simulink model "TwoSegmentArm_muscles"  (R2024b)
settings: Solver=VariableStepAuto  StartTime=0.0  StopTime=5  RelTol=1e-3  AbsTol=1e-3  EnableMultiTasking=on
model workspace (MAT data in the model file):
  bp_out = [-2.4 1.9]
values from neighbouring files (symbols this model uses):
  Param_Mus_MEE = Library_mtu_simulink_mtu_standard_parameters(Param_Mus_MEE)    [init_muscle_MEE.m]
  Param_Mus_MEF = Library_mtu_simulink_mtu_standard_parameters(Param_Mus_MEF)    [init_muscle_MEF.m]
  Param_Mus_MSA = Library_mtu_simulink_mtu_standard_parameters(Param_Mus_MSA)    [init_muscle_MSA.m]
  Param_Mus_MSR = Library_mtu_simulink_mtu_standard_parameters(Param_Mus_MSR)    [init_muscle_MSR.m]
  random_offset = 0    [ddpg_agent.m]
  Ts = 0.075    [ddpg_agent.m]
undefined symbols (not defined in the file or in its folder): DiscIntNeverNeededParam, gaussian, X, Y, Z
libraries: sm_lib x25, nesl_utility x15, simulink x10, Library_mtu_simulink x8, rllib x1
(part 1 of 2)
settings Model: Creator=Isabell  LastModifiedBy=morit
settings SolverCC: AutoScaleAbsTol=off  AlgebraicLoopSolver=TrustRegion
settings DataIOCC: LimitDataPoints=on  MaxDataPoints=10000
settings OptimizationCC: LifeSpan=inf
settings DebuggingCC: UnconnectedInputMsg=warning  UnconnectedOutputMsg=warning  UnconnectedLineMsg=warning  AllowSymbolicDim=off  SFUnexpectedBacktrackingDiag=warning  SFNoUnconditionalDefaultTransitionDiag=warning  SFExecutionAtInitializationDiag=none  ArithmeticOperatorsInVariantConditions=warning
settings ModelReferenceCC: EnableRefExpFcnMdlSchedulingChecks=on
settings SFSimCC: SimUseLocalCustomCode=off  CustomCodeUndefinedFunction=UseInterfaceOnly
settings RTWCC: RTWUseLocalCustomCode=off  GPUComputeCapability=3.5  DLArmComputeVersion=19.05
settings CodeAppCC: StateflowObjectComments=on
settings GRTTargetCC: TargetLangStandard=C89/C90 (ANSI)
settings ConfigComp: CovMetricSettings=dw  CovSaveCumulativeToWorkspaceVar=on  CovSaveSingleToWorkspaceVar=on  CovExternalEMLEnable=off  CovSFcnEnable=off
settings SimscapeCC: SimscapeLogType=all  SimscapeLogSimulationStatistics=on  SimscapeLogDataHistory=10000

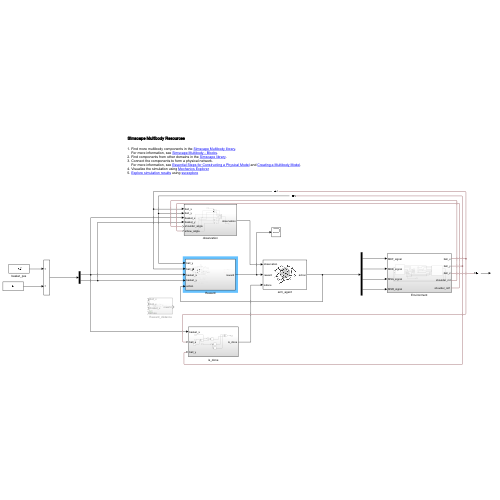
[thumbnail: Simulink's stored preview of the top-level diagram]
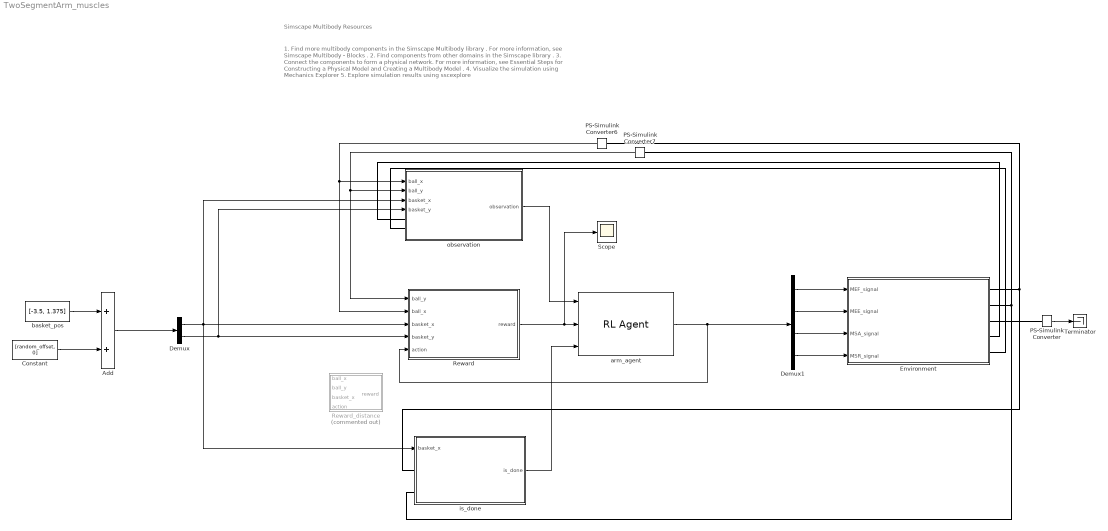
== system TwoSegmentArm_muscles ==
  note: 1. Find more multibody components in the Simscape Multibody library .
      | For more information, see Simscape Multibody - Blocks .
      | 2. Find components from other domains in the Simscape library .
      | 3. Connect the components to form a physical network.
      | For more information, see Essential Steps for Constructing a Physical Model and Creating a Multibody Model .
      | 4. Visualize the simulation using Mechanics Explorer
      | 5. Explore simulation results using sscexplore
  note: Simscape Multibody Resources
  Add : Sum
  Constant : Constant  Value=[random_offset, 0]
  Demux : Demux  Outputs=2
  Demux1 : Demux
  Environment : Subsystem
  PS-Simulink Converter : nesl_utility/PS-Simulink Converter  PhysicalDomain=network_engine_domain  SubClassName=ps_output  LeftPortType=input  RightPortType=output  PseudoPeriodic=off  Frequencies=[]  VectorFormat=inherit  Unit=inherit  AffineConversion=off
  PS-Simulink Converter6 : nesl_utility/PS-Simulink Converter  PhysicalDomain=network_engine_domain  SubClassName=ps_output  LeftPortType=input  RightPortType=output  PseudoPeriodic=off  Frequencies=[]  VectorFormat=inherit  Unit=inherit  AffineConversion=off
  PS-Simulink Converter7 : nesl_utility/PS-Simulink Converter  PhysicalDomain=network_engine_domain  SubClassName=ps_output  LeftPortType=input  RightPortType=output  PseudoPeriodic=off  Frequencies=[]  VectorFormat=inherit  Unit=inherit  AffineConversion=off
  Reward : Subsystem
  Reward_distance : Subsystem  Commented=on
  Scope : Scope
  Terminator : Terminator
  arm_agent : rllib/RL Agent  Agent=agent  ExternalActionAsInput=off  ProvideLastAction=off  ProvideCumRwd=off  TreatAsDirectFeedthrough=on  UseStrictObservationDataTypes=off
  basket_pos : Constant  Value=[-3.5, 1.375]
  is_done : Subsystem
  observation : Subsystem
  wires:
  basket_pos/1 -> Add/1
  Add/1 -> Demux/1
  Demux1/3 -> Environment/3(MSA_signal)
  Demux1/2 -> Environment/2(MEE_signal)
  Constant/1 -> Add/2
  Demux1/1 -> Environment/1(MEF_signal)
  Demux1/4 -> Environment/4(MSR_signal)
  PS-Simulink Converter/1 -> Terminator/1
  observation/1(observation) -> arm_agent/1
  Demux/2 -> observation/4(basket_y), Reward/4(basket_y)
  Demux/1 -> Reward/3(basket_x), observation/3(basket_x), is_done/1(basket_x)
  is_done/1(is_done) -> arm_agent/3
  Reward/1(reward) -> Scope/1, arm_agent/2
  PS-Simulink Converter7/1 -> observation/2(ball_y), Reward/1(ball_y)
  arm_agent/1 -> Reward/5(action), Demux1/1
  PS-Simulink Converter6/1 -> Reward/2(ball_x), observation/1(ball_x)
  connections:
  Environment/RConn3 -- PS-Simulink Converter/LConn1
  Environment/RConn5 -- observation/LConn2
  Environment/RConn4 -- observation/LConn1
  Environment/RConn1 -- PS-Simulink Converter6/LConn1 -- is_done/LConn1
  PS-Simulink Converter7/LConn1 -- is_done/LConn2 -- Environment/RConn2

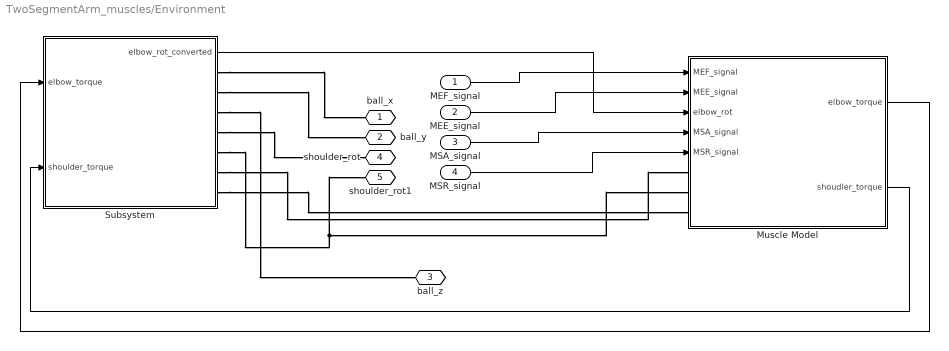
== system TwoSegmentArm_muscles/Environment ==
  MEF_signal : Inport
  MEE_signal : Inport  Port=2
  MSA_signal : Inport  Port=3
  MSR_signal : Inport  Port=4
  Muscle Model : Subsystem
  Subsystem : Subsystem
  ball_x : PMIOPort  Side=Right
  ball_y : PMIOPort  Port=2  Side=Right
  ball_z : PMIOPort  Port=3  Side=Right
  shoulder_rot : PMIOPort  Port=4  Side=Right
  shoulder_rot1 : PMIOPort  Port=5  Side=Right
  wires:
  Muscle Model/2(shoudler_torque) -> Subsystem/2(shoulder_torque)
  Subsystem/1(elbow_rot_converted) -> Muscle Model/3(elbow_rot)
  MEF_signal/1 -> Muscle Model/1(MEF_signal)
  Muscle Model/1(elbow_torque) -> Subsystem/1(elbow_torque)
  MSA_signal/1 -> Muscle Model/4(MSA_signal)
  MSR_signal/1 -> Muscle Model/5(MSR_signal)
  MEE_signal/1 -> Muscle Model/2(MEE_signal)
  connections:
  Subsystem/RConn7 -- Muscle Model/LConn3
  Subsystem/RConn5 -- shoulder_rot1/RConn1 -- Muscle Model/LConn2
  Subsystem/RConn3 -- ball_z/RConn1
  Subsystem/RConn2 -- ball_y/RConn1
  Subsystem/RConn6 -- Muscle Model/LConn1
  Subsystem/RConn1 -- ball_x/RConn1
  Subsystem/RConn4 -- shoulder_rot/RConn1

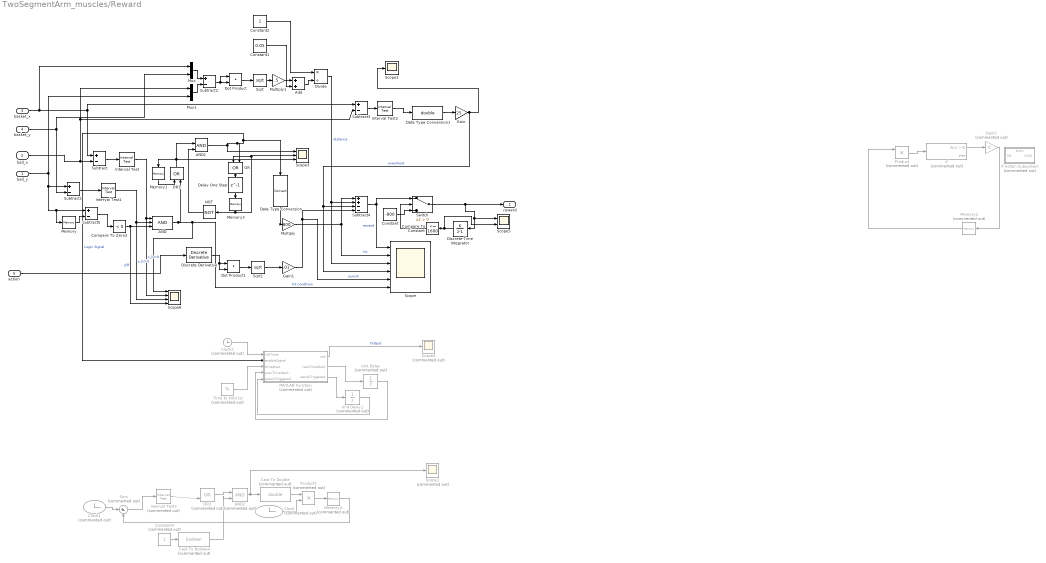
== system TwoSegmentArm_muscles/Reward ==
  ball_y : Inport
  ball_x : Inport  Port=2
  basket_x : Inport  Port=3
  basket_y : Inport  Port=4
  action : Inport  Port=5
  AND : Logic  Inputs=3  IconShape=distinctive  AllPortsSameDT=off  OutDataTypeStr=boolean
  AND1 : Logic  IconShape=distinctive  AllPortsSameDT=off  OutDataTypeStr=boolean
  AND2 : Logic  Commented=on  IconShape=distinctive  AllPortsSameDT=off  OutDataTypeStr=boolean
  Add : Sum
  Cast To Boolean : DataTypeConversion  Commented=on  OutDataTypeStr=boolean  SaturateOnIntegerOverflow=off  RndMeth=Floor
  Cast To Double : DataTypeConversion  Commented=on  OutDataTypeStr=double  SaturateOnIntegerOverflow=off  RndMeth=Floor
  Clock : Clock  Commented=on
  Clock1 : Clock  Commented=on
  Clock2 : Clock  Commented=on
  Compare To Constant : simulink/Logic and Bit Operations/Compare To Constant  relop=<=  const=1600  OutDataTypeStr=uint8
  Compare To Zero2 : simulink/Logic and Bit Operations/Compare To Zero  relop=<  OutDataTypeStr=boolean
  Constant : Constant  Value=-800
  Constant1 : Constant  Value=0.05
  Constant2 : Constant
  Constant4 : Constant  Commented=on
  Data Type Conversion : DataTypeConversion  SaturateOnIntegerOverflow=off  RndMeth=Floor
  Data Type Conversion1 : DataTypeConversion  OutDataTypeStr=double  SaturateOnIntegerOverflow=off  RndMeth=Floor
  Delay One Step : Delay  DelayLength=1  SampleTime=Ts * 0.985
  Discrete Derivative : simulink/Discrete/Discrete Derivative  gainval=1.0  ICPrevScaledInput=0.0  OutMin=[]  OutMax=[]  OutDataType=fixdt(1, 16)  OutScaling=2^-10  DoSatur=off
  Discrete-Time Integrator : DiscreteIntegrator  IntegratorMethod=Accumulation: Forward Euler  SampleTime=Ts  ICPrevOutput=DiscIntNeverNeededParam  ICPrevScaledInput=DiscIntNeverNeededParam
  Divide : Product  Inputs=*/
  Dot Product : DotProduct  OutDataTypeStr=Inherit: Inherit via internal rule
  Dot Product1 : DotProduct  OutDataTypeStr=Inherit: Inherit via internal rule
  Gain : Gain  Gain=25
  Gain1 : Gain  Gain=.01
  Gain2 : Gain  Commented=on  Gain=0
  If : If  Commented=on
  If Action Subsystem : Subsystem  Commented=on  TreatAsAtomicUnit=on
  Interval Test : simulink/Logic and Bit Operations/Interval Test  IntervalClosedRight=on  uplimit=0.225  IntervalClosedLeft=on  lowlimit=-0.225  OutDataTypeStr=boolean
  Interval Test1 : simulink/Logic and Bit Operations/Interval Test  IntervalClosedRight=on  uplimit=0.05  IntervalClosedLeft=on  lowlimit=-0.35  OutDataTypeStr=boolean
  Interval Test2 : simulink/Logic and Bit Operations/Interval Test  IntervalClosedRight=on  uplimit=0.85  IntervalClosedLeft=on  lowlimit=0.25  OutDataTypeStr=boolean
  Interval Test3 : simulink/Logic and Bit Operations/Interval Test  Commented=on  IntervalClosedRight=on  uplimit=Ts  IntervalClosedLeft=on  lowlimit=0  OutDataTypeStr=boolean
  MATLAB Function : MATLAB Function  Commented=on  TreatAsAtomicUnit=on
  Memory : Memory
  Memory1 : Memory
  Memory2 : Memory  Commented=on
  Memory3 : Memory
  Memory4 : Memory  Commented=on  InitialCondition=-1
  Multiply : Gain  Gain=800
  Multiply1 : Gain  Gain=.5
  Mux : Mux  Inputs=2
  Mux1 : Mux  Inputs=2
  NOT : Logic  Operator=NOT  IconShape=distinctive  AllPortsSameDT=off  OutDataTypeStr=boolean
  OR : Logic  Operator=OR  IconShape=distinctive  AllPortsSameDT=off  OutDataTypeStr=boolean
  OR1 : Logic  Operator=OR  IconShape=distinctive  AllPortsSameDT=off  OutDataTypeStr=boolean
  OR2 : Logic  Commented=on  Operator=OR  IconShape=distinctive  AllPortsSameDT=off  OutDataTypeStr=boolean
  Product : Product  Commented=on
  Product1 : Product  Commented=on
  Scope : Scope  NumInputPorts=6
  Scope1 : Scope  Commented=on
  Scope2 : Scope
  Scope3 : Scope  NumInputPorts=3
  Scope4 : Scope  Commented=on
  Scope5 : Scope  NumInputPorts=2
  Scope6 : Scope  NumInputPorts=4
  Sqrt : Sqrt
  Sqrt1 : Sqrt
  Subtract{,1..3,5} (5 alike) : Sum  Inputs=+-
  Subtract4 : Sum  Inputs=++--
  Sum : Sum  Commented=on  Inputs=|+-
  Switch : Switch  Criteria=u2 > Threshold  SaturateOnIntegerOverflow=off  InputSameDT=off
  Time to hold (s) : Constant  Commented=on  Value=Ts
  Unit Delay : UnitDelay  Commented=on  SampleTime=-1  HasFrameUpgradeWarning=on
  Unit Delay1 : UnitDelay  Commented=on  SampleTime=-1  HasFrameUpgradeWarning=on
  reward : Outport
  wires:
  basket_x/1 -> Subtract3/1, Subtract/1, Mux/1
  ball_x/1 -> Mux1/1, Subtract3/2, Subtract/2
  Subtract/1 -> Interval Test/1
  ball_y/1 -> Subtract1/1, Memory/1, Subtract5/1, Mux1/2
  Subtract5/1 -> Compare To Zero2/1
  basket_y/1 -> Mux/2, Subtract1/2
  Divide/1 -> Scope/3, Subtract4/2  "distance"
  Subtract4/1 -> Scope/1, Switch/1  "reward"
  Interval Test/1 -> Scope6/2, AND/1  "x_limit"
  Subtract1/1 -> Interval Test1/1
  Interval Test1/1 -> Scope6/3, AND/2  "y_limit"
  Mux/1 -> Subtract2/1
  Mux1/1 -> Subtract2/2
  Subtract2/1 -> Dot Product/2, Dot Product/1
  Dot Product/1 -> Sqrt/1
  Sqrt/1 -> Multiply1/1
  Subtract3/1 -> Interval Test2/1
  Interval Test2/1 -> Data Type Conversion1/1
  Data Type Conversion1/1 -> Gain/1
  Gain/1 -> Scope/4, Subtract4/3, Scope2/1  "overshoot"
  Dot Product1/1 -> Sqrt1/1
  Gain1/1 -> Scope/5, Subtract4/4  "punish"
  Constant2/1 -> Divide/1
  Multiply1/1 -> Add/1
  Sqrt1/1 -> Gain1/1
  Compare To Zero2/1 -> Scope6/4, AND/3  "diff"
  Memory/1 -> Subtract5/2
  action/1 -> Discrete Derivative/1
  Discrete Derivative/1 -> Dot Product1/2, Dot Product1/1
  Add/1 -> Divide/2
  Constant1/1 -> Add/2
  AND/1 -> Scope6/1, Scope/6, OR1/2  "hit condition"
  Memory2/1 -> Product/1
  Gain2/1 -> Memory2/1
  If/1 -> Gain2/1
  Product/1 -> If/1
  ? -> Product/2
  Multiply/1 -> Subtract4/1, Scope/2  "hit"
  NOT/1 -> AND1/2
  Clock/1 -> Product1/2
  Cast To Double/1 -> Product1/1
  Product1/1 -> Memory4/1
  Memory4/1 -> Sum/2
  Clock1/1 -> Sum/1
  Interval Test3/1 -> OR2/2
  AND2/1 -> Scope1/1, Cast To Double/1
  OR2/1 -> AND2/1
  Constant4/1 -> Cast To Boolean/1
  Cast To Boolean/1 -> AND2/2
  Sum/1 -> Interval Test3/1
  Time to hold (s)/1 -> MATLAB Function/3(timeWait)
  AND1/1 -> Data Type Conversion/1, MATLAB Function/2(enableSignal), OR/2, Scope3/1  "Logic Signal"
  Clock2/1 -> MATLAB Function/1(clkTime)
  MATLAB Function/1(out) -> Scope4/1  "Output"
  MATLAB Function/2(newTimeStart) -> Unit Delay/1
  MATLAB Function/3(newIsTriggered) -> Unit Delay1/1
  Unit Delay1/1 -> MATLAB Function/5(prevIsTriggered)
  Unit Delay/1 -> MATLAB Function/4(prevTimeStart)
  Data Type Conversion/1 -> Multiply/1
  OR/1 -> Delay One Step/1
  Memory3/1 -> Scope3/2, OR/1, NOT/1
  OR1/1 -> AND1/1, Memory1/1, Scope3/3
  Memory1/1 -> OR1/1
  Delay One Step/1 -> Memory3/1
  Switch/1 -> Discrete-Time Integrator/1, Scope5/1, reward/1
  Constant/1 -> Switch/3
  Discrete-Time Integrator/1 -> Scope5/2, Compare To Constant/1
  Compare To Constant/1 -> Switch/2

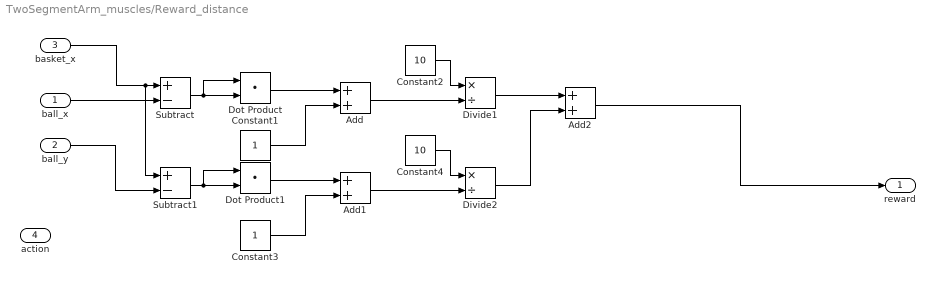
== system TwoSegmentArm_muscles/Reward_distance ==
  ball_x : Inport
  ball_y : Inport  Port=2
  basket_x : Inport  Port=3
  action : Inport  Port=4
  Add : Sum
  Add1 : Sum
  Add2 : Sum
  Constant1 : Constant
  Constant2 : Constant  Value=10
  Constant3 : Constant
  Constant4 : Constant  Value=10
  Divide1 : Product  Inputs=*/
  Divide2 : Product  Inputs=*/
  Dot Product : DotProduct  OutDataTypeStr=Inherit: Inherit via internal rule
  Dot Product1 : DotProduct  OutDataTypeStr=Inherit: Inherit via internal rule
  Subtract : Sum  Inputs=+-
  Subtract1 : Sum  Inputs=+-
  reward : Outport
  wires:
  Add/1 -> Divide1/2
  Constant2/1 -> Divide1/1
  Subtract/1 -> Dot Product/1, Dot Product/2
  ball_x/1 -> Subtract/2
  Dot Product/1 -> Add/1
  Constant1/1 -> Add/2
  basket_x/1 -> Subtract1/1, Subtract/1
  Divide1/1 -> Add2/1
  Add1/1 -> Divide2/2
  Constant4/1 -> Divide2/1
  Dot Product1/1 -> Add1/1
  Subtract1/1 -> Dot Product1/1, Dot Product1/2
  Constant3/1 -> Add1/2
  Add2/1 -> reward/1
  Divide2/1 -> Add2/2
  ball_y/1 -> Subtract1/2

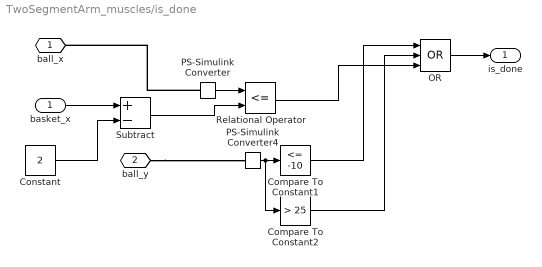
== system TwoSegmentArm_muscles/is_done ==
  basket_x : Inport
  Compare To Constant1 : simulink/Logic and Bit Operations/Compare To Constant  relop=<=  const=-10  OutDataTypeStr=boolean
  Compare To Constant2 : simulink/Logic and Bit Operations/Compare To Constant  relop=>  const=25  OutDataTypeStr=boolean
  Constant : Constant  Value=2
  OR : Logic  Operator=OR  Inputs=3  IconShape=distinctive  AllPortsSameDT=off  OutDataTypeStr=boolean
  PS-Simulink Converter : nesl_utility/PS-Simulink Converter  PhysicalDomain=network_engine_domain  SubClassName=ps_output  LeftPortType=input  RightPortType=output  PseudoPeriodic=off  Frequencies=[]  VectorFormat=inherit  Unit=inherit  AffineConversion=off
  PS-Simulink Converter4 : nesl_utility/PS-Simulink Converter  PhysicalDomain=network_engine_domain  SubClassName=ps_output  LeftPortType=input  RightPortType=output  PseudoPeriodic=off  Frequencies=[]  VectorFormat=inherit  Unit=inherit  AffineConversion=off
  Relational Operator : RelationalOperator  Operator=<=  OutDataTypeStr=boolean  RndMeth=Simplest  InputSameDT=off
  Subtract : Sum  Inputs=+-
  ball_x : PMIOPort  Side=Left
  ball_y : PMIOPort  Port=2  Side=Left
  is_done : Outport
  wires:
  PS-Simulink Converter4/1 -> Compare To Constant2/1, Compare To Constant1/1
  Compare To Constant1/1 -> OR/1
  Compare To Constant2/1 -> OR/2
  OR/1 -> is_done/1
  PS-Simulink Converter/1 -> Relational Operator/1
  Relational Operator/1 -> OR/3
  Constant/1 -> Subtract/2
  Subtract/1 -> Relational Operator/2
  basket_x/1 -> Subtract/1
  connections:
  ball_y/RConn1 -- PS-Simulink Converter4/LConn1
  PS-Simulink Converter/LConn1 -- ball_x/RConn1

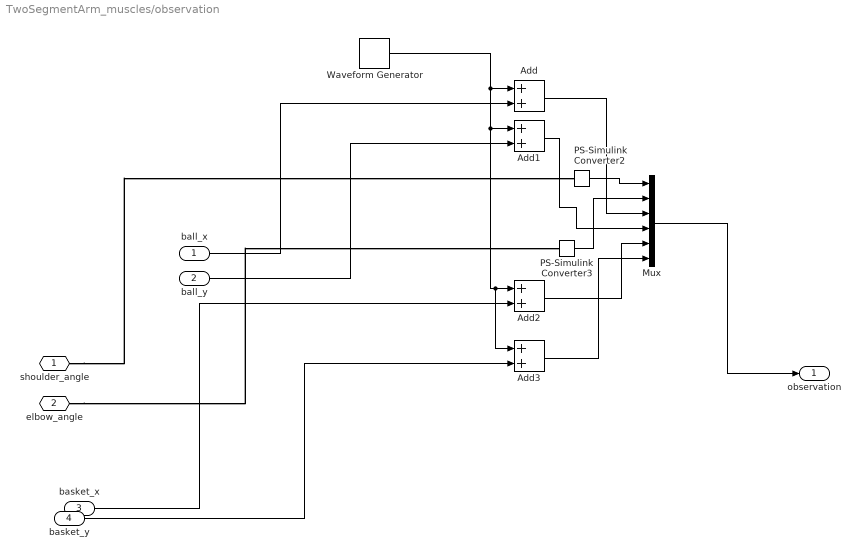
== system TwoSegmentArm_muscles/observation ==
  ball_x : Inport
  ball_y : Inport  Port=2
  basket_x : Inport  Port=3
  basket_y : Inport  Port=4
  Add{,1..3} (4 alike) : Sum
  Mux : Mux  Inputs=6
  PS-Simulink Converter2 : nesl_utility/PS-Simulink Converter  PhysicalDomain=network_engine_domain  SubClassName=ps_output  LeftPortType=input  RightPortType=output  PseudoPeriodic=off  Frequencies=[]  VectorFormat=inherit  Unit=inherit  AffineConversion=off
  PS-Simulink Converter3 : nesl_utility/PS-Simulink Converter  PhysicalDomain=network_engine_domain  SubClassName=ps_output  LeftPortType=input  RightPortType=output  PseudoPeriodic=off  Frequencies=[]  VectorFormat=inherit  Unit=inherit  AffineConversion=off
  Waveform Generator : simulink/Sources/Waveform Generator  OutMin=[]  OutMax=[]  OutDataTypeStr=double  SelectedSignal=1  Signals=gaussian(0, 0, 120)  BlockNames=MultiportSwitch_2798d07791aa46f  SampleTime=0.1
  shoulder_angle : PMIOPort  Side=Left
  elbow_angle : PMIOPort  Port=2  Side=Left
  observation : Outport
  wires:
  Add/1 -> Mux/3
  Add1/1 -> Mux/4
  Waveform Generator/1 -> Add3/1, Add2/1, Add1/1, Add/1
  PS-Simulink Converter3/1 -> Mux/2
  Add3/1 -> Mux/6
  PS-Simulink Converter2/1 -> Mux/1
  Add2/1 -> Mux/5
  basket_y/1 -> Add3/2
  ball_x/1 -> Add/2
  Mux/1 -> observation/1
  ball_y/1 -> Add1/2
  basket_x/1 -> Add2/2
  connections:
  elbow_angle/RConn1 -- PS-Simulink Converter3/LConn1
  shoulder_angle/RConn1 -- PS-Simulink Converter2/LConn1

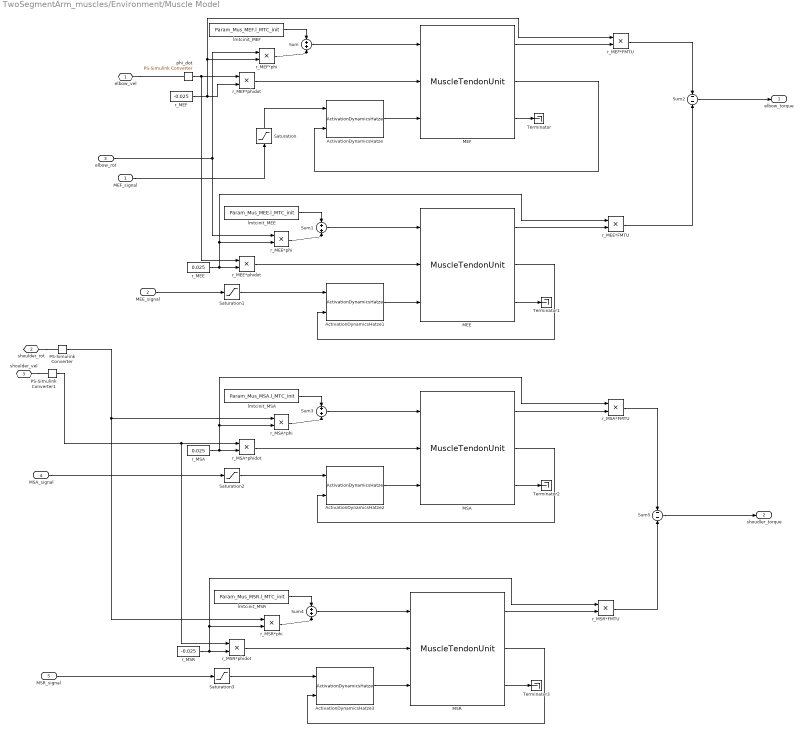
== system TwoSegmentArm_muscles/Environment/Muscle Model ==
  MEF_signal : Inport
  MEE_signal : Inport  Port=2
  elbow_rot : Inport  Port=3
  MSA_signal : Inport  Port=4
  MSR_signal : Inport  Port=5
  ActivationDynamicsHatze : Library_mtu_simulink/ActivationDynamicsHatze  Act_Param=Param_Mus_MEF.ActDyn  Mus_Param=Param_Mus_MEF
  ActivationDynamicsHatze1 : Library_mtu_simulink/ActivationDynamicsHatze  Act_Param=Param_Mus_MEE.ActDyn  Mus_Param=Param_Mus_MEE
  ActivationDynamicsHatze2 : Library_mtu_simulink/ActivationDynamicsHatze  Act_Param=Param_Mus_MEE.ActDyn  Mus_Param=Param_Mus_MEE
  ActivationDynamicsHatze3 : Library_mtu_simulink/ActivationDynamicsHatze  Act_Param=Param_Mus_MEE.ActDyn  Mus_Param=Param_Mus_MEE
  MEE : Library_mtu_simulink/MuscleTendonUnit  Mus_Param=Param_Mus_MEE
  MEF : Library_mtu_simulink/MuscleTendonUnit  Mus_Param=Param_Mus_MEF
  MSA : Library_mtu_simulink/MuscleTendonUnit  Mus_Param=Param_Mus_MSA
  MSR : Library_mtu_simulink/MuscleTendonUnit  Mus_Param=Param_Mus_MSR
  PS-Simulink Converter : nesl_utility/PS-Simulink Converter  PhysicalDomain=network_engine_domain  SubClassName=ps_output  LeftPortType=input  RightPortType=output  PseudoPeriodic=off  Frequencies=[]  VectorFormat=inherit  Unit=inherit  AffineConversion=off
  PS-Simulink Converter1 : nesl_utility/PS-Simulink Converter  PhysicalDomain=network_engine_domain  SubClassName=ps_output  LeftPortType=input  RightPortType=output  PseudoPeriodic=off  Frequencies=[]  VectorFormat=inherit  Unit=inherit  AffineConversion=off
  Saturation{,1..3} (4 alike) : Saturate  UpperLimit=1  LowerLimit=0
  Sum{,1,3..4} (4 alike) : Sum  Inputs=+|+
  Sum2 : Sum  Inputs=-|-
  Sum5 : Sum  Inputs=-|-
  Terminator{,1..3} (4 alike) : Terminator
  lmtcinit_MEE : Constant  Value=Param_Mus_MEE.l_MTC_init
  lmtcinit_MEF : Constant  Value=Param_Mus_MEF.l_MTC_init
  lmtcinit_MSA : Constant  Value=Param_Mus_MSA.l_MTC_init
  lmtcinit_MSR : Constant  Value=Param_Mus_MSR.l_MTC_init
  phi_dot : nesl_utility/PS-Simulink Converter  PhysicalDomain=network_engine_domain  SubClassName=ps_output  LeftPortType=input  RightPortType=output  PseudoPeriodic=off  Frequencies=[]  VectorFormat=1-D array  Unit=inherit  AffineConversion=off
  r_MEE : Constant  Value=0.025
  r_MEE*FMTU : Product
  r_MEE*phi : Product
  r_MEE*phidot : Product
  r_MEF : Constant  Value=-0.025
  r_MEF*FMTU : Product
  r_MEF*phi : Product
  r_MEF*phidot : Product
  r_MSA : Constant  Value=0.025
  r_MSA*FMTU : Product
  r_MSA*phi : Product
  r_MSA*phidot : Product
  r_MSR : Constant  Value=-0.025
  r_MSR*FMTU : Product
  r_MSR*phi : Product
  r_MSR*phidot : Product
  elbow_vel : PMIOPort  Side=Left
  shoulder_rot : PMIOPort  Port=2  Side=Left
  shoulder_vel : PMIOPort  Port=3  Side=Left
  elbow_torque : Outport
  shoudler_torque : Outport  Port=2
  wires:
  Sum1/1 -> MEE/1
  MEE/3 -> Terminator1/1
  r_MEE*phi/1 -> Sum1/2
  elbow_rot/1 -> r_MEF*phi/1, r_MEE*phi/1
  r_MEF*phi/1 -> Sum/2
  r_MEF*phidot/1 -> MEF/2
  r_MEE/1 -> r_MEE*FMTU/1, r_MEE*phi/2, r_MEE*phidot/2
  MEF/3 -> Terminator/1
  r_MEE*FMTU/1 -> Sum2/2
  Saturation/1 -> ActivationDynamicsHatze/1
  MEE/1 -> r_MEE*FMTU/2
  r_MEF/1 -> r_MEF*FMTU/1, r_MEF*phi/2, r_MEF*phidot/2
  ActivationDynamicsHatze/1 -> MEF/3
  ActivationDynamicsHatze1/1 -> MEE/3
  Saturation1/1 -> ActivationDynamicsHatze1/1
  MEF/2 -> ActivationDynamicsHatze/2
  Sum/1 -> MEF/1
  MEF/1 -> r_MEF*FMTU/2
  MEE_signal/1 -> Saturation1/1
  phi_dot/1 -> r_MEE*phidot/1, r_MEF*phidot/1
  lmtcinit_MEF/1 -> Sum/1
  r_MEF*FMTU/1 -> Sum2/1
  r_MEE*phidot/1 -> MEE/2
  lmtcinit_MEE/1 -> Sum1/1
  MEE/2 -> ActivationDynamicsHatze1/2
  Sum2/1 -> elbow_torque/1
  MEF_signal/1 -> Saturation/1
  MSR/2 -> ActivationDynamicsHatze3/2
  MSR/1 -> r_MSR*FMTU/2
  r_MSR*FMTU/1 -> Sum5/2
  PS-Simulink Converter/1 -> r_MSR*phi/1, r_MSA*phi/1
  r_MSR*phi/1 -> Sum4/2
  PS-Simulink Converter1/1 -> r_MSR*phidot/1, r_MSA*phidot/1
  MSR/3 -> Terminator3/1
  ActivationDynamicsHatze3/1 -> MSR/3
  ActivationDynamicsHatze2/1 -> MSA/3
  Saturation3/1 -> ActivationDynamicsHatze3/1
  r_MSA*phidot/1 -> MSA/2
  r_MSR/1 -> r_MSR*FMTU/1, r_MSR*phi/2, r_MSR*phidot/2
  r_MSA*phi/1 -> Sum3/2
  Sum4/1 -> MSR/1
  MSA/2 -> ActivationDynamicsHatze2/2
  Sum3/1 -> MSA/1
  r_MSA*FMTU/1 -> Sum5/1
  Saturation2/1 -> ActivationDynamicsHatze2/1
  r_MSR*phidot/1 -> MSR/2
  MSA/3 -> Terminator2/1
  lmtcinit_MSR/1 -> Sum4/1
  lmtcinit_MSA/1 -> Sum3/1
  r_MSA/1 -> r_MSA*FMTU/1, r_MSA*phi/2, r_MSA*phidot/2
  MSA/1 -> r_MSA*FMTU/2
  MSA_signal/1 -> Saturation2/1
  MSR_signal/1 -> Saturation3/1
  Sum5/1 -> shoudler_torque/1
  connections:
  elbow_vel/RConn1 -- phi_dot/LConn1
  shoulder_rot/RConn1 -- PS-Simulink Converter/LConn1
  shoulder_vel/RConn1 -- PS-Simulink Converter1/LConn1
